simulink model "sampled_communication"  (R2025b)
settings: Solver=ode4  StartTime=0.0  StopTime=10  FixedStep=0.01  RelTol=1e-3
model workspace (MAT data in the model file):
  delay_s = Simulink.Parameter
  delay_s.Value = 0.1
  delay_s.Complexity = 'real'
  delay_s.Dimensions = [1 1]
  delay_s.DataType = 'double'
  delay_s.DocUnits = 's'
  sample_period_s = Simulink.Parameter
  sample_period_s.Value = 0.05
  sample_period_s.Complexity = 'real'
  sample_period_s.Dimensions = [1 1]
  sample_period_s.DataType = 'double'
  sample_period_s.DocUnits = 's'
settings Model: ParameterArgumentNames=sample_period_s,delay_s  Creator=miyut  LastModifiedBy=miyut
settings DataIOCC: SaveOutput=off  SignalLogging=off

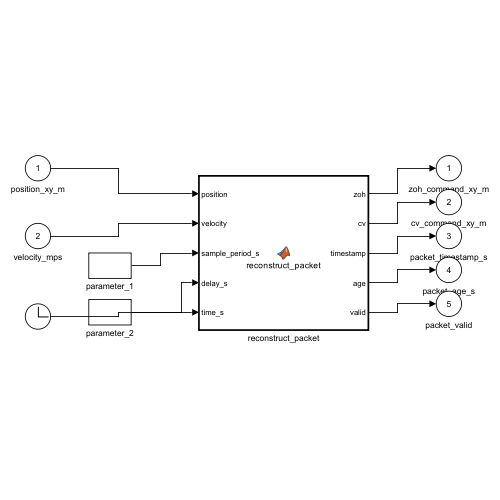
[thumbnail: Simulink's stored preview of the top-level diagram]
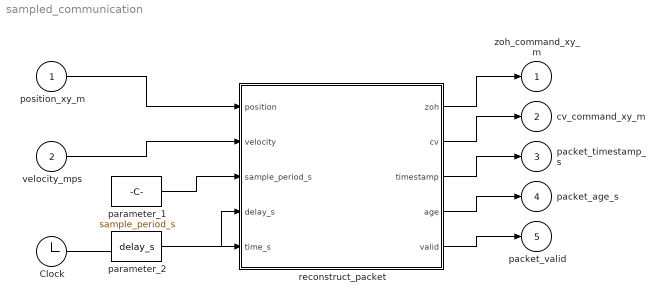
== system sampled_communication ==
  position_xy_m : Inport  OutDataTypeStr=double  Unit=m  PortDimensions=2
  velocity_mps : Inport  Port=2  OutDataTypeStr=double  Unit=m/s  PortDimensions=2
  Clock : Clock
  parameter_1 : Constant  Value=sample_period_s
  parameter_2 : Constant  Value=delay_s
  reconstruct_packet : MATLAB Function  TreatAsAtomicUnit=on
  zoh_command_xy_m : Outport  OutDataTypeStr=double  Unit=m  PortDimensions=2
  cv_command_xy_m : Outport  Port=2  OutDataTypeStr=double  Unit=m  PortDimensions=2
  packet_timestamp_s : Outport  Port=3  OutDataTypeStr=double  Unit=s  PortDimensions=1
  packet_age_s : Outport  Port=4  OutDataTypeStr=double  Unit=s  PortDimensions=1
  packet_valid : Outport  Port=5  OutDataTypeStr=boolean  PortDimensions=1
  wires:
  position_xy_m/1 -> reconstruct_packet/1(position)
  velocity_mps/1 -> reconstruct_packet/2(velocity)
  Clock/1 -> reconstruct_packet/5(time_s)
  parameter_1/1 -> reconstruct_packet/3(sample_period_s)
  parameter_2/1 -> reconstruct_packet/4(delay_s)
  reconstruct_packet/1(zoh) -> zoh_command_xy_m/1
  reconstruct_packet/2(cv) -> cv_command_xy_m/1
  reconstruct_packet/3(timestamp) -> packet_timestamp_s/1
  reconstruct_packet/4(age) -> packet_age_s/1
  reconstruct_packet/5(valid) -> packet_valid/1

== matlab function sampled_communication/reconstruct_packet ==
  data: position input double size=[1 2]; zoh output double size=[1 2]; velocity input double size=[1 2]; sample_period_s input double size=1; delay_s input double size=1; time_s input double size=1; cv output double size=[1 2]; timestamp output double size=1; age output double size=1; valid output boolean size=1
function [zoh, cv, timestamp, age, valid] = reconstruct_packet(position, velocity, sample_period_s, delay_s, time_s)
%#codegen
persistent next_sample write_index packet_count packet_timestamps packet_positions packet_velocities
buffer_capacity = 1024.0;
if isempty(packet_count)
    next_sample = 0.0; write_index = 1.0; packet_count = 0.0;
    packet_timestamps = -ones(1,buffer_capacity); packet_positions = zeros(buffer_capacity,2); packet_velocities = zeros(buffer_capacity,2);
end
tol = 1.0e-10;
if ~(isfinite(sample_period_s) && sample_period_s > 0.0)
    error('teleopDelay:InvalidSamplePeriod', 'sample_period_s must be positive and finite.');
end
if ~(isfinite(delay_s) && delay_s >= 0.0)
    error('teleopDelay:InvalidDelay', 'delay_s must be nonnegative and finite.');
end
if time_s + tol >= next_sample
    packet_timestamps(write_index) = next_sample; packet_positions(write_index,:) = position; packet_velocities(write_index,:) = velocity;
    write_index = write_index + 1.0; if write_index > buffer_capacity, write_index = 1.0; end; packet_count = min(packet_count + 1.0, buffer_capacity);
    next_sample = next_sample + sample_period_s;
end
selected_timestamp = -1.0; selected_position = zeros(1,2); selected_velocity = zeros(1,2); selected_valid = false;
for index = 1:buffer_capacity
    if index <= packet_count && packet_timestamps(index) + delay_s <= time_s + tol && packet_timestamps(index) > selected_timestamp
        selected_timestamp = packet_timestamps(index); selected_position = packet_positions(index,:); selected_velocity = packet_velocities(index,:); selected_valid = true;
    end
end
if selected_valid
    valid = true; timestamp = selected_timestamp; age = max(0.0, time_s - selected_timestamp); zoh = selected_position; cv = selected_position + age * selected_velocity;
else
    valid = false; timestamp = 0.0; age = 0.0; zoh = zeros(1,2); cv = zeros(1,2);
end
end
